simulink model "BESS_test"  (Simulink 8.8)
settings: Solver=ode1  StartTime=0.0  StopTime=15  FixedStep=Ts  MaxStep=1e-3  RelTol=1e-3  EnableMultiTasking=on
model workspace (MAT data in the model file):
  op_snapshot1 : opcond.OperatingPoint (value not decoded)
values from neighbouring files (symbols this model uses):
  dPer = 0.05    [Software_BESS_init.m]
  f = 60    [Software_BESS_init.m]
  filt = firstOrderDig(50e-3, Tc, 'low')    [Software_BESS_init.m]    (also in firstOrderDig.m = (tau*s) / (tau*s + 1))
  H = 2    [Software_BESS_init.m]
  Igrid = Pgrid/Vgrid/3    [Software_BESS_init.m]
  Lgrid = (Zgrid/2)/(2*pi*f)    [Software_BESS_init.m]
  paramDroopFreq2Reac = 0.5*(1/dPer)    (= 10)    [Software_BESS_init.m]
  paramDroopFreq2Real = 0*(1/dPer)    (= 0)    [Software_BESS_init.m]
  paramDroopVolts2Reac = 0*(1/dPer)    (= 0)    [Software_BESS_init.m]
  paramDroopVolts2Real = 0.5*(1/dPer)    (= 10)    [Software_BESS_init.m]
  Pgrid = 3e6    (= 3000000)    [Software_BESS_init.m]
  Rgrid = Zgrid/2    [Software_BESS_init.m]
  sys_mech = ss(1/(tau_mech*s+1))    [Software_BESS_init.m]
  Tc = Ts    (= 0.0001)    [Software_BESS_init.m]
  Ts = 100e-6    (= 0.0001)    [Software_BESS_init.m]
  Vdc_nom = 1000    [Software_BESS_init.m]
  Vgrid = 480/sqrt(3)    [Software_BESS_init.m]
undefined symbols (not defined in the file or in its folder): BESS, BESS_lib, DiscIntNeverNeededParam, RotatingMachine_lib, VSource
undefined symbols (not defined in the file): batt_esr, batt_kWh
libraries: powerlib x29, simulink x7, powerlib_meascontrol x6, transformer_lib x4, breaker_lib x3, Load_lib x3, cables_lib x2, IsourcePower_lib x1
settings Model: ARTEMISmethode_block_infos=$$__separator__$$RS/ARTEMIS Guide$$__separator__$$  Creator=RE25624  LastModifiedBy=ch24070
settings SolverCC: ZeroCrossAlgorithm=Adaptive
settings DataIOCC: ExternalInput=getinputstruct(op_snapshot1)  InitialState=getstatestruct(op_snapshot1)  LimitDataPoints=off  MaxDataPoints=90060  SignalLoggingSaveFormat=Dataset  SaveOutput=off  SignalLogging=off  DSMLogging=off  SaveTime=off  OutputSaveName=result
settings OptimizationCC: BlockReduction=off  OptimizeBlockIOStorage=off  BufferReuse=off  GlobalBufferReuse=off  ExpressionFolding=off  ExpressionDepthLimit=2147483647  LocalBlockOutputs=off  EfficientMapNaN2IntZero=off
settings DebuggingCC: MaxConsecutiveZCsMsg=warning  IgnoredZcDiagnostic=none  MultiTaskRateTransMsg=warning  UnconnectedLineMsg=none  ModelReferenceExtraNoncontSigs=warning
settings HardwareCC: TargetBitPerPointer=64  TargetBitPerSizeT=64  TargetBitPerPtrDiffT=64  TargetLongLongMode=on  TargetIntDivRoundTo=Zero  TargetEndianess=LittleEndian  TargetWordSize=64  TargetHWDeviceType=MATLAB Host  ProdEqTarget=off
settings ModelReferenceCC: UpdateModelReferenceTargets=IfOutOfDate
settings SFSimCC: SFSimEcho=off
settings CodeAppCC: MaxIdLength=128
settings GRTTargetCC: GeneratePreprocessorConditionals=Use local settings

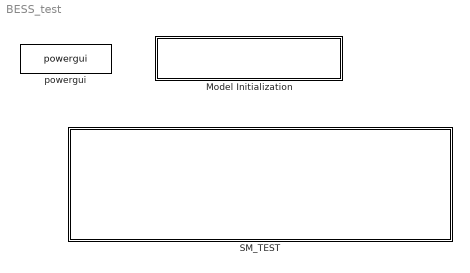
== system BESS_test ==
  Model Initialization : Subsystem  AncestorBlock=artemis/Tools /Misc/Model Initialization  mask(Model Functions){InitFcnX=, prel=off, posl=on, inif=on, strf=off}
      mask prompts: InitFcnX "Initialisation"; prel "Preload Function"; posl "PostLoad Function"; inif "InitFcn"; strf "StartFcn"
      mask init:
      | currentBlock = gcb;
      | root = bdroot(currentBlock);
      | 
      | if ~strcmp(get_param(root,'BlockDiagramType'),'library')
      |     if prel==1
      |         set_param(root, 'PreLoadFcn', InitFcnX);
      |     else
      |         set_param(root, 'PreLoadFcn', '');
      |     end
      |     if inif==1
      |         set_param(root, 'InitFcn', InitFcnX);
      |     else
      |         set_param(root, 'InitFcn', '');
      |     end
      |     if strf==1
      |         set_param(root, 'StartFcn', InitFcnX);
      |     else
      |         set_param(root, 'StartFcn', '');
      |     end
      |     if posl==1
      |         set_param(root, 'PostLoadFcn', InitFcnX);
      |     else
      |         set_param(root, 'PostLoadFcn', '');
      |     end
      | end
      | 
      | pos = get_param(currentBlock, 'Position');
      | width = pos(3) - pos(1); height = pos(4) - pos(2);
      | txt = [ upper(root) '\n' '- InitFcn. . . . . '  get_param(root, 'InitFcn') ];
      settings: CopyFcn=set_param(gcb,'LinkStatus','inactive')
      mask Display: text(5, height*0.5, txt, 'horizontalAlignment', 'left', 'verticalAlignment', 'middle') ;
  SM_TEST : Subsystem
  powergui : powerlib/powergui  Priority=2  SimulationMode=Discrete  SolverType=Tustin  SampleTime=Ts  frequency=60  SPID=off  DisableSnubberDevices=off  DisableRonSwitches=off  DisableVfSwitches=off  SwTol=0  DisplayEquations=off  Interpol=off  ExternalGateDelay=off  methode=off  Ts=0  FunctionMessages=off  echomessages=off  HookPort=off  EnableUseOfTLC=off  x0status=blocks  frequencyindice=0  Pbase=100e6  ErrMax=1e-4  Iterations=50  UnitsV=kV  UnitsW=MW  buscounter=0  RestoreLinks=warning  ResistiveCurrentMeasurement=off  Frange=logspace(-2,3,50)  Ylog=on  Xlog=on  ShowGrid=off  save=off  variable=ZData  structure=0  ZoomFFT=on  StartTime=0.0  cycles=2  DisplayStyle=off  fundamental=60  FreqAxis=off  MaxFrequency=1000  frequencyindicesteady=1  RmsSteady=1  display=off

== system BESS_test/Model Initialization ==

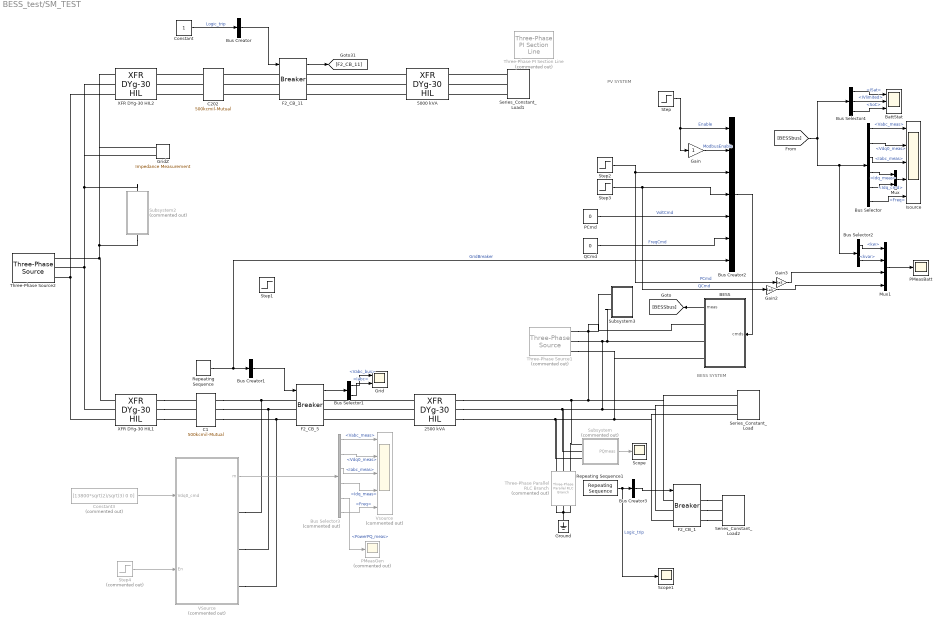
== system BESS_test/SM_TEST ==
  note: PV SYSTEM
  note: BESS SYSTEM
  2500 kVA : transformer_lib/XFR DYg-30 HIL  Rating=2500  Vp=13800  Vs=480  Z=5.56  XR=5.52
  5000 kVA : transformer_lib/XFR DYg-30 HIL  Rating=5000  Vp=13800  Vs=480  Z=5.50  XR=5.44
  BESS : Subsystem  AncestorBlock=BESS_lib/BESS
  BattStat : Scope  NumInputPorts=3
  Bus Creator : BusCreator  Inputs=1
  Bus Creator1 : BusCreator  Inputs=1
  Bus Creator2 : BusCreator  Inputs=7
  Bus Creator3 : BusCreator  Inputs=1
  Bus Selector : BusSelector  OutputSignals=Inverter.Vabc_meas,Inverter.Vdq0_meas,Inverter.Iabc_meas,Inverter.Idq_meas,Inverter.Idq_cmd,Inverter.Freq
  Bus Selector1 : BusSelector  OutputSignals=Vabc_bus,Iabc
  Bus Selector2 : BusSelector  OutputSignals=Inverter.kw,Inverter.kvar
  Bus Selector3 : BusSelector  Commented=on  OutputSignals=Vabc_meas,Vdq0_meas,Iabc_meas,Idq_meas,PowerPQ_meas,Freq
  Bus Selector4 : BusSelector  OutputSignals=Inverter.faults.ISat,Inverter.faults.IVlimited,Battery.SoC
  C1 : cables_lib/500kcmil-Mutual  length=2000  par_sets=1  ratio=3
  C202 : cables_lib/500kcmil-Mutual  length=2000  par_sets=1  ratio=3
  Constant : Constant
  Constant3 : Constant  Commented=on  Value=[13800*sqrt(2)/sqrt(3) 0 0]
  F2_CB_1 : breaker_lib/Breaker  Ts=Ts  mech_delay=3/60
  F2_CB_11 : breaker_lib/Breaker  Ts=Ts  mech_delay=3/60
  F2_CB_5 : breaker_lib/Breaker  Ts=Ts  mech_delay=3/60
  Gain : Gain
  Gain2 : Gain  Gain=1e3
  Gain3 : Gain  Gain=1e3
  Grid : Scope  NumInputPorts=2
  GridZ : powerlib/Measurements/Impedance Measurement  LConnTagsString=+|-  Factor=1
  Ground : powerlib/Elements/Ground  LConnTagsString=a
  Isource : Scope  NumInputPorts=5
  Mux : Mux  Inputs=2
  Mux1 : Mux
  PCmd : Constant  Value=0
  PMeasBatt : Scope
  PMeasGen : Scope  Commented=on
  QCmd : Constant  Value=0
  Repeating Sequence : simulink/Sources/Repeating Sequence  rep_seq_t=[0 2 2+Ts 6 6+Ts 100]  rep_seq_y=[1 1 0 0 1 1]
  Repeating Sequence1 : simulink/Sources/Repeating Sequence  rep_seq_t=[0, 4, 4+Ts, 5, 5+Ts, 8, 8+Ts 20]  rep_seq_y=[0 0 1 1 0 0 1 1]
  Scope : Scope
  Scope1 : Scope
  Series_Constant_Load : Load_lib/Series_Constant_Load  v=460  kVA=400  pf=0.90
  Series_Constant_Load1 : Load_lib/Series_Constant_Load  v=460  kVA=100  pf=0.90
  Series_Constant_Load2 : Load_lib/Series_Constant_Load  v=460  kVA=300  pf=0.90
  Step : Step  Time=0.2  SampleTime=0
  Step1 : Step  Time=0.5  Before=1  After=0  SampleTime=0
  Step2 : Step  Time=9  After=-500  SampleTime=0
  Step3 : Step  Time=13  After=-500  SampleTime=0
  Step4 : Step  Commented=on  Time=0  SampleTime=0
  Subsystem : Subsystem  Commented=on  mask{V=480, P=1e3, PF=0.9}
      mask prompts: V "Nominal voltage LL"; P "P (kVA)"
      mask init:
      | Rpar = V^2/(P*1e3*PF)
      | Lpar = (V^2/((P*1e3*sqrt(1-PF^2))/3))/377
      | if Lpar == Inf
      |     Lser=0
      |     Rser=Rpar
      | else
      |     Lser = 1e-3
      |     Rser = (-Lpar^2)/(Rpar+Lpar)+Lpar-Lser
      | end
  Subsystem2 : Subsystem  Commented=on
  Subsystem3 : Subsystem
  Three-Phase PI Section Line : powerlib/Elements/Three-Phase PI Section Line  Commented=on  LConnTagsString=a|b|c  RConnTagsString=A|B|C  Frequency=60  Resistances=[ 0.01273 0.3864]  Inductances="[ 0.9337e-3  4.1264e-3]"  Capacitances=[12.74e-9 7.751e-9]  Length=100
  Three-Phase Parallel RLC Branch : powerlib/Elements/Three-Phase Parallel RLC Branch  Commented=on  LConnTagsString=A|B|C  RConnTagsString=A|B|C  BranchType=R  Resistance=Vgrid^2/(200*1e3/3);  Inductance=(Vgrid^2/((1000e3*sqrt(1-0.9^2))/3))/377  Capacitance=1e-6  Measurements=None
  Three-Phase Source1 : powerlib/Electrical Sources/Three-Phase Source  Commented=on  InternalConnection=Yg  VoltagePhases=off  Voltage=480  PhaseAngle=0  Voltage_phases=[25e3 25e3 25e3]/sqrt(3)  PhaseAngles_phases=[0 -120 +120]  Frequency=60  NonIdealSource=on  SpecifyImpedance=off  Resistance=Lgrid  Inductance=Rgrid  ShortCircuitLevel=2000e6  BaseVoltage=480  XRratio=100  BusType=swing  Pref=0  Qref=0  Prefabc=[10e3, 10e3, 10e3]  Qrefabc=[0, 0, 0]  Qmin=-inf  Qmax=inf
  Three-Phase Source2 : powerlib/Electrical Sources/Three-Phase Source  InternalConnection=Yg  VoltagePhases=off  Voltage=115000  PhaseAngle=0  Voltage_phases=[25e3 25e3 25e3]/sqrt(3)  PhaseAngles_phases=[0 -120 +120]  Frequency=60  NonIdealSource=on  SpecifyImpedance=on  Resistance=0.8929  Inductance=16.58e-3  ShortCircuitLevel=2000e6  BaseVoltage=115000  XRratio=100  BusType=swing  Pref=0  Qref=0  Prefabc=[10e3, 10e3, 10e3]  Qrefabc=[0, 0, 0]  Qmin=-inf  Qmax=inf
  VSource : Subsystem  Commented=on  AncestorBlock=RotatingMachine_lib/VSource
  Vsource : Scope  Commented=on  NumInputPorts=5
  XFR DYg-30 HIL1 : transformer_lib/XFR DYg-30 HIL  Rating=50000  Vp=115000  Vs=13800  Z=6  XR=30
  XFR DYg-30 HIL2 : transformer_lib/XFR DYg-30 HIL  Rating=50000  Vp=115000  Vs=13800  Z=6  XR=30
  wires:
  F2_CB_5/1 -> Bus Selector1/1
  F2_CB_11/1 -> [F2_CB_11]
  Constant/1 -> Bus Creator/1  "Logic_trip"
  Repeating Sequence/1 -> Bus Creator2/7, Bus Creator1/1  "GridBreaker"
  Bus Creator1/1 -> F2_CB_5/1
  Bus Creator/1 -> F2_CB_11/1
  Step/1 -> Bus Creator2/1, Gain/1  "Enable"
  Step2/1 -> Bus Creator2/3, Gain3/1  "PCmd"
  Step3/1 -> Bus Creator2/4, Gain2/1  "QCmd"
  Bus Creator2/1 -> BESS/1(cmds)
  Bus Selector/6 -> Isource/5  "<Freq>"
  Bus Selector/3 -> Isource/3  "<Iabc_meas>"
  Bus Selector/1 -> Isource/1  "<Vabc_meas>"
  Bus Selector/2 -> Isource/2  "<Vdq0_meas>"
  Subsystem/1(PQmeas) -> Scope/1
  Bus Selector1/1 -> Grid/1  "<Vabc_bus>"
  Bus Selector1/2 -> Grid/2  "<Iabc>"
  Mux/1 -> Isource/4
  Bus Selector/4 -> Mux/1  "<Idq_meas>"
  Bus Selector/5 -> Mux/2  "<Idq_cmd>"
  BESS/1(meas) -> [BESSbus]
  [BESSbus] -> Bus Selector/1, Bus Selector2/1, Bus Selector4/1
  Bus Selector2/1 -> Mux1/1  "<kw>"
  Mux1/1 -> PMeasBatt/1
  Repeating Sequence1/1 -> Scope1/1, Bus Creator3/1  "Logic_trip"
  Bus Creator3/1 -> F2_CB_1/1
  Gain2/1 -> Mux1/4
  Gain3/1 -> Mux1/3
  Constant3/1 -> VSource/1(Vdq0_cmd)
  Step4/1 -> VSource/2(En)
  Bus Selector3/3 -> Vsource/3  "<Iabc_meas>"
  Bus Selector3/1 -> Vsource/1  "<Vabc_meas>"
  Bus Selector3/2 -> Vsource/2  "<Vdq0_meas>"
  Bus Selector3/4 -> Vsource/4  "<Idq_meas>"
  VSource/1(m) -> Bus Selector3/1
  Bus Selector3/6 -> Vsource/5  "<Freq>"
  Bus Selector3/5 -> PMeasGen/1  "<PowerPQ_meas>"
  Gain/1 -> Bus Creator2/2  "ModbusEnable"
  Bus Selector2/2 -> Mux1/2  "<kvar>"
  Bus Selector4/2 -> BattStat/2  "<IVlimited>"
  Bus Selector4/1 -> BattStat/1  "<ISat>"
  Bus Selector4/3 -> BattStat/3  "<SoC>"
  PCmd/1 -> Bus Creator2/5  "VoltCmd"
  QCmd/1 -> Bus Creator2/6  "FreqCmd"
  connections:
  5000 kVA/LConn2 -- F2_CB_11/RConn2
  2500 kVA/LConn1 -- F2_CB_5/RConn1
  2500 kVA/LConn3 -- F2_CB_5/RConn3
  2500 kVA/LConn2 -- F2_CB_5/RConn2
  5000 kVA/LConn1 -- F2_CB_11/RConn1
  5000 kVA/LConn3 -- F2_CB_11/RConn3
  2500 kVA/RConn1 -- BESS/RConn1 -- Subsystem3/LConn1 -- Three-Phase Source1/RConn1 -- F2_CB_1/LConn1 -- Series_Constant_Load/LConn1 -- Three-Phase Parallel RLC Branch/LConn3 -- Subsystem/LConn1
  2500 kVA/RConn3 -- BESS/RConn3 -- Three-Phase Source1/RConn3 -- F2_CB_1/LConn3 -- Series_Constant_Load/LConn3 -- Three-Phase Parallel RLC Branch/LConn1 -- Subsystem/LConn3
  XFR DYg-30 HIL1/LConn1 -- GridZ/LConn1 -- XFR DYg-30 HIL2/LConn1 -- Subsystem2/LConn1 -- Three-Phase Source2/RConn1
  XFR DYg-30 HIL1/LConn2 -- GridZ/LConn2 -- XFR DYg-30 HIL2/LConn2 -- Subsystem2/RConn1 -- Three-Phase Source2/RConn2
  XFR DYg-30 HIL1/LConn3 -- XFR DYg-30 HIL2/LConn3 -- Three-Phase Source2/RConn3
  Series_Constant_Load1/LConn3 -- 5000 kVA/RConn3
  Series_Constant_Load1/LConn2 -- 5000 kVA/RConn2
  Series_Constant_Load1/LConn1 -- 5000 kVA/RConn1
  C202/LConn1 -- XFR DYg-30 HIL2/RConn1
  C202/LConn2 -- XFR DYg-30 HIL2/RConn2
  C202/LConn3 -- XFR DYg-30 HIL2/RConn3
  XFR DYg-30 HIL1/RConn1 -- C1/LConn1
  XFR DYg-30 HIL1/RConn2 -- C1/LConn2
  XFR DYg-30 HIL1/RConn3 -- C1/LConn3
  C1/RConn2 -- VSource/RConn2 -- F2_CB_5/LConn2
  C1/RConn1 -- VSource/RConn1 -- F2_CB_5/LConn1
  C1/RConn3 -- VSource/RConn3 -- F2_CB_5/LConn3
  F2_CB_11/LConn1 -- C202/RConn1
  F2_CB_11/LConn2 -- C202/RConn2
  F2_CB_11/LConn3 -- C202/RConn3
  Ground/LConn1 -- Three-Phase Parallel RLC Branch/RConn3 -- Three-Phase Parallel RLC Branch/RConn1 -- Three-Phase Parallel RLC Branch/RConn2
  F2_CB_1/RConn1 -- Series_Constant_Load2/LConn1
  F2_CB_1/RConn2 -- Series_Constant_Load2/LConn2
  F2_CB_1/RConn3 -- Series_Constant_Load2/LConn3
  Subsystem3/LConn2 -- BESS/RConn2 -- 2500 kVA/RConn2 -- Three-Phase Parallel RLC Branch/LConn2 -- Subsystem/LConn2 -- F2_CB_1/LConn2 -- Series_Constant_Load/LConn2 -- Three-Phase Source1/RConn2

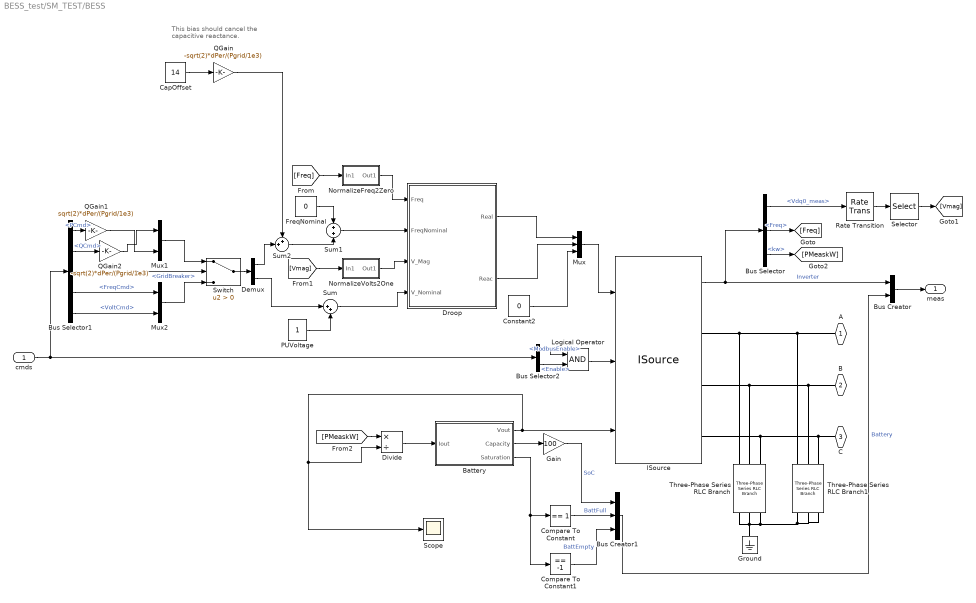
== system BESS_test/SM_TEST/BESS ==
  note: This bias should cancel
      | the capacitive reactance.
  cmds : Inport
  Battery : Subsystem  mask(Very simple battery model.){kWh=batt_kWh, esr=batt_esr, Vdc_nom=Vdc_nom}
      mask prompts: kWh "Capacity  (kWh)"; esr "Output Resistance (Ohms)"; Vdc_nom "Open Circuit Voltage"
      mask help: Model integrates charge and stops at the rated capacity. When charge is all removed the current drops to zero.
      mask Help: This model views the battery as a voltage source with a fixed equivalent series resistance and a perfect integrator for capacity.
  Bus Creator : BusCreator  Inputs=2
  Bus Creator1 : BusCreator  Inputs=3
  Bus Selector : BusSelector  OutputSignals=Vdq0_meas,Freq,kw
  Bus Selector1 : BusSelector  OutputSignals=PCmd,QCmd,GridBreaker,FreqCmd,VoltCmd
  Bus Selector2 : BusSelector  OutputSignals=ModbusEnable,Enable
  CapOffset : Constant  Value=14
  Compare To Constant : simulink/Logic and Bit Operations/Compare To Constant  relop===  const=1  OutDataTypeStr=boolean
  Compare To Constant1 : simulink/Logic and Bit Operations/Compare To Constant  relop===  const=-1  OutDataTypeStr=boolean
  Constant2 : Constant  Value=0
  Demux : Demux  Outputs=2
  Divide : Product  Inputs=*/
  Droop : Subsystem
  FreqNominal : Constant  Value=0
  Gain : Gain  Gain=100
  Ground : powerlib/Elements/Ground  LConnTagsString=a
  ISource : IsourcePower_lib/ISource
  Logical Operator : Logic  AllPortsSameDT=off  OutDataTypeStr=boolean
  Mux : Mux  Inputs=3
  Mux1 : Mux  Inputs=2
  Mux2 : Mux  Inputs=2
  NormalizeFreq2Zero : Subsystem
  NormalizeVolts2One : Subsystem
  PUVoltage : Constant
  QGain : Gain  Gain=-sqrt(2)*dPer/(Pgrid/1e3)
  QGain1 : Gain  Gain=sqrt(2)*dPer/(Pgrid/1e3)
  QGain2 : Gain  Gain=-sqrt(2)*dPer/(Pgrid/1e3)
  Rate Transition : RateTransition  OutPortSampleTime=Tc
  Scope : Scope
  Selector : Selector  InputPortWidth=3  IndexOptions=Index vector (dialog)  Indices=[1]  OutputSizes=1
  Sum : Sum  Inputs=|++
  Sum1 : Sum
  Sum2 : Sum  Inputs=++|
  Switch : Switch  Criteria=u2 > Threshold
  Three-Phase Series RLC Branch : powerlib/Elements/Three-Phase Series RLC Branch  LConnTagsString=A|B|C  RConnTagsString=A|B|C  BranchType=RC  Resistance=10e-3  Inductance=1e-3  Capacitance=1e-3  Measurements=None
  Three-Phase Series RLC Branch1 : powerlib/Elements/Three-Phase Series RLC Branch  LConnTagsString=A|B|C  RConnTagsString=A|B|C  BranchType=R  Resistance=10000  Inductance=1e-3  Capacitance=1000e-9  Measurements=None
  A : PMIOPort  Port=1  Side=Right
  B : PMIOPort  Port=2  Side=Right
  C : PMIOPort  Port=3  Side=Right
  meas : Outport
  wires:
  ISource/1 -> Bus Creator/1, Bus Selector/1  "Inverter"
  cmds/1 -> Bus Selector2/1, Bus Selector1/1
  FreqNominal/1 -> Sum1/1
  Sum/1 -> Droop/4(V_Nominal)
  PUVoltage/1 -> Sum/2
  Sum1/1 -> Droop/2(FreqNominal)
  Constant2/1 -> Mux/3
  [Freq] -> NormalizeFreq2Zero/1(In1)
  Mux/1 -> ISource/1
  Selector/1 -> [Vmag]
  Bus Selector/1 -> Rate Transition/1  "<Vdq0_meas>"
  Bus Selector/2 -> [Freq]  "<Freq>"
  Rate Transition/1 -> Selector/1
  Droop/1(Real) -> Mux/1
  Droop/2(Reac) -> Mux/2
  NormalizeFreq2Zero/1(Out1) -> Droop/1(Freq)
  NormalizeVolts2One/1(Out1) -> Droop/3(V_Mag)
  [Vmag] -> NormalizeVolts2One/1(In1)
  Sum2/1 -> Sum1/2
  QGain/1 -> Sum2/1
  CapOffset/1 -> QGain/1
  Bus Selector2/2 -> Logical Operator/2  "<Enable>"
  Bus Selector2/1 -> Logical Operator/1  "<ModbusEnable>"
  Logical Operator/1 -> ISource/2
  Bus Selector/3 -> [PMeaskW]  "<kw>"
  [PMeaskW] -> Divide/1
  Divide/1 -> Battery/1(Iout)
  Battery/1(Vout) -> ISource/3, Scope/1, Divide/2
  Bus Creator/1 -> meas/1
  Gain/1 -> Bus Creator1/1  "SoC"
  Battery/2(Capacity) -> Gain/1
  Compare To Constant/1 -> Bus Creator1/2  "BattFull"
  Battery/3(Saturation) -> Compare To Constant1/1, Compare To Constant/1
  Compare To Constant1/1 -> Bus Creator1/3  "BattEmpty"
  Bus Creator1/1 -> Bus Creator/2  "Battery"
  Bus Selector1/3 -> Switch/2  "<GridBreaker>"
  Switch/1 -> Demux/1
  Demux/1 -> Sum2/2
  Demux/2 -> Sum/1
  Mux2/1 -> Switch/3
  Bus Selector1/1 -> QGain1/1  "<PCmd>"
  Bus Selector1/2 -> QGain2/1  "<QCmd>"
  Bus Selector1/4 -> Mux2/1  "<FreqCmd>"
  Bus Selector1/5 -> Mux2/2  "<VoltCmd>"
  Mux1/1 -> Switch/1
  QGain1/1 -> Mux1/2
  QGain2/1 -> Mux1/1
  connections:
  Three-Phase Series RLC Branch/LConn1 -- Three-Phase Series RLC Branch1/LConn1 -- A/RConn1 -- ISource/RConn1
  Three-Phase Series RLC Branch/LConn3 -- Three-Phase Series RLC Branch1/LConn3 -- C/RConn1 -- ISource/RConn3
  Three-Phase Series RLC Branch/LConn2 -- Three-Phase Series RLC Branch1/LConn2 -- B/RConn1 -- ISource/RConn2
  Ground/LConn1 -- Three-Phase Series RLC Branch1/RConn3 -- Three-Phase Series RLC Branch1/RConn2 -- Three-Phase Series RLC Branch1/RConn1 -- Three-Phase Series RLC Branch/RConn3 -- Three-Phase Series RLC Branch/RConn1 -- Three-Phase Series RLC Branch/RConn2

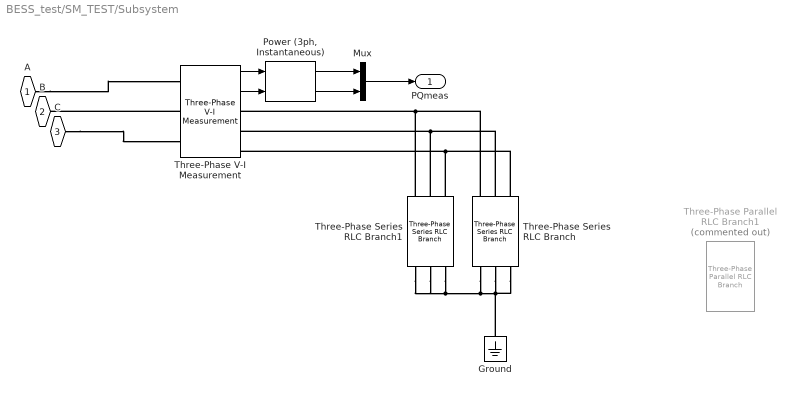
== system BESS_test/SM_TEST/Subsystem ==
  Ground : powerlib/Elements/Ground  LConnTagsString=a
  Mux : Mux  Inputs=2
  "Power (3ph, Instantaneous)" : powerlib_meascontrol/Measurements/Power (3ph, Instantaneous)
  Three-Phase Parallel RLC Branch1 : powerlib/Elements/Three-Phase Parallel RLC Branch  Commented=on  LConnTagsString=A|B|C  RConnTagsString=A|B|C  BranchType=RL  Resistance=Vgrid^2/(1000e3*0.9/3)  Inductance=(Vgrid^2/((1000e3*sqrt(1-0.9^2))/3))/377  Capacitance=1e-6  Measurements=None
  Three-Phase Series RLC Branch : powerlib/Elements/Three-Phase Series RLC Branch  LConnTagsString=A|B|C  RConnTagsString=A|B|C  BranchType=L  Resistance=Rser  Inductance=Lpar  Capacitance=1e-6  Measurements=None
  Three-Phase Series RLC Branch1 : powerlib/Elements/Three-Phase Series RLC Branch  LConnTagsString=A|B|C  RConnTagsString=A|B|C  BranchType=R  Resistance=Rpar  Inductance=Lser  Capacitance=1e-6  Measurements=None
  Three-Phase V-I Measurement : powerlib/Measurements/Three-Phase V-I Measurement  VoltageMeasurement=phase-to-ground  SetLabelV=off  LabelV=Vabc  Vpu=off  VpuLL=off  CurrentMeasurement=yes  SetLabelI=off  LabelI=Iabc  Ipu=off  Pbase=100e6  Vbase=500e3  OutputType=Complex  PhasorSimulation=off  PSBequivalent=0
  A : PMIOPort  Port=1  Side=Left
  B : PMIOPort  Port=2  Side=Left
  C : PMIOPort  Port=3  Side=Left
  PQmeas : Outport
  wires:
  Three-Phase V-I Measurement/1 -> "Power (3ph, Instantaneous)"/1
  Three-Phase V-I Measurement/2 -> "Power (3ph, Instantaneous)"/2
  "Power (3ph, Instantaneous)"/1 -> Mux/1
  "Power (3ph, Instantaneous)"/2 -> Mux/2
  Mux/1 -> PQmeas/1
  connections:
  Three-Phase V-I Measurement/LConn2 -- B/RConn1
  C/RConn1 -- Three-Phase V-I Measurement/LConn3
  A/RConn1 -- Three-Phase V-I Measurement/LConn1
  Three-Phase Series RLC Branch/LConn1 -- Three-Phase Series RLC Branch1/LConn1 -- Three-Phase V-I Measurement/RConn1
  Three-Phase Series RLC Branch/LConn2 -- Three-Phase Series RLC Branch1/LConn2 -- Three-Phase V-I Measurement/RConn2
  Three-Phase Series RLC Branch/LConn3 -- Three-Phase Series RLC Branch1/LConn3 -- Three-Phase V-I Measurement/RConn3
  Ground/LConn1 -- Three-Phase Series RLC Branch1/RConn3 -- Three-Phase Series RLC Branch1/RConn2 -- Three-Phase Series RLC Branch1/RConn1 -- Three-Phase Series RLC Branch/RConn1 -- Three-Phase Series RLC Branch/RConn2 -- Three-Phase Series RLC Branch/RConn3

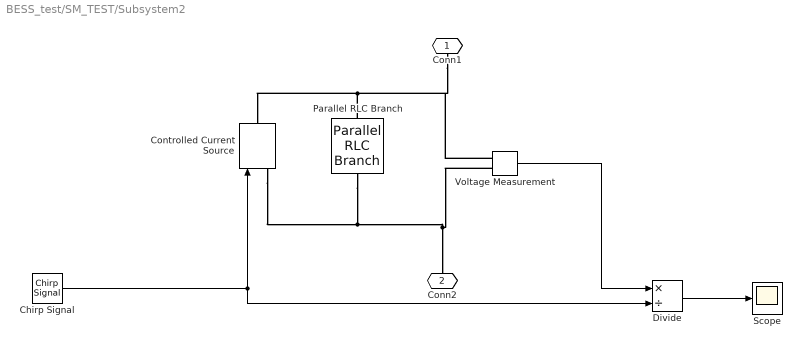
== system BESS_test/SM_TEST/Subsystem2 ==
  Chirp Signal : simulink/Sources/Chirp Signal  f1=0.1  T=1  f2=1000
  Controlled Current Source : powerlib/Electrical Sources/Controlled Current Source  Initialize=on  Source_Type=AC  Amplitude=0  Phase=0  Frequency=0  Measurements=None
  Divide : Product  Inputs=*/
  Parallel RLC Branch : powerlib/Elements/Parallel RLC Branch  LConnTagsString=a  RConnTagsString=__new0  BranchType=R  Resistance=1e6  Inductance=1e-3  SetiL0=off  InitialCurrent=0  Capacitance=1e-6  Setx0=off  InitialVoltage=0  Measurements=None
  Scope : Scope
  Voltage Measurement : powerlib/Measurements/Voltage Measurement  PhasorSimulation=off  OutputType=Complex  PSBequivalent=0
  Conn1 : PMIOPort  Port=1  Side=Right
  Conn2 : PMIOPort  Port=2  Side=Left
  wires:
  Chirp Signal/1 -> Divide/2, Controlled Current Source/1
  Voltage Measurement/1 -> Divide/1
  Divide/1 -> Scope/1
  connections:
  Controlled Current Source/LConn1 -- Parallel RLC Branch/RConn1 -- Voltage Measurement/LConn2 -- Conn2/RConn1
  Parallel RLC Branch/LConn1 -- Conn1/RConn1 -- Voltage Measurement/LConn1 -- Controlled Current Source/RConn1

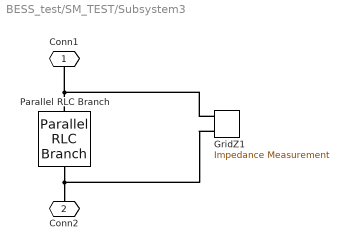
== system BESS_test/SM_TEST/Subsystem3 ==
  GridZ1 : powerlib/Measurements/Impedance Measurement  LConnTagsString=+|-  Factor=1
  Parallel RLC Branch : powerlib/Elements/Parallel RLC Branch  LConnTagsString=a  RConnTagsString=__new0  BranchType=R  Resistance=1e6  Inductance=1e-3  SetiL0=off  InitialCurrent=0  Capacitance=1e-6  Setx0=off  InitialVoltage=0  Measurements=None
  Conn1 : PMIOPort  Port=1  Side=Left
  Conn2 : PMIOPort  Port=2  Side=Left
  connections:
  GridZ1/LConn1 -- Parallel RLC Branch/LConn1 -- Conn1/RConn1
  GridZ1/LConn2 -- Parallel RLC Branch/RConn1 -- Conn2/RConn1

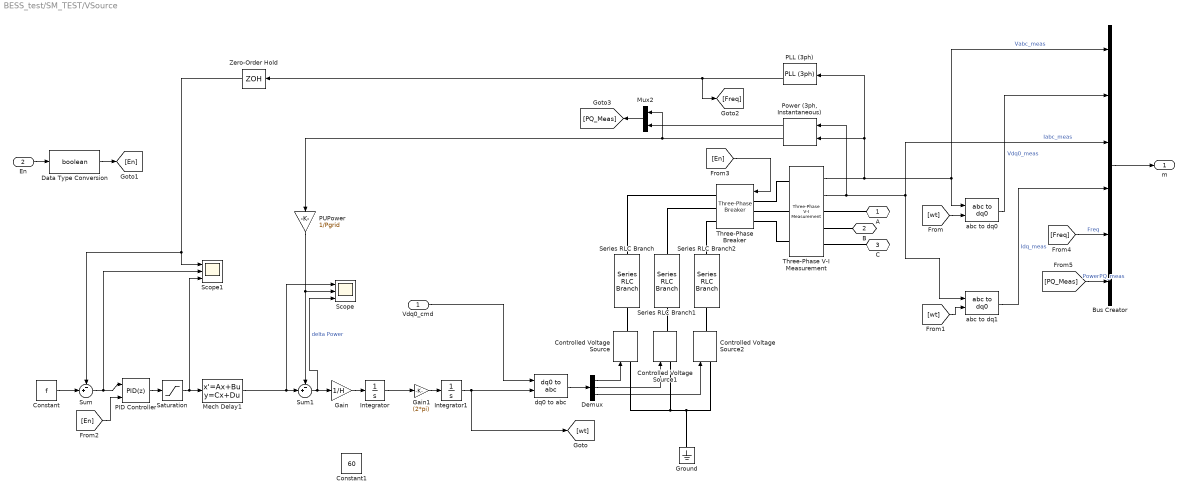
== system BESS_test/SM_TEST/VSource ==
  Vdq0_cmd : Inport
  En : Inport  Port=2
  Bus Creator : BusCreator  Inputs=6
  Constant : Constant  Value=f
  Constant1 : Constant  Value=60
  Controlled Voltage Source : powerlib/Electrical Sources/Controlled Voltage Source  Initialize=on  Source_Type=AC  Amplitude=0  Phase=0  Frequency=0  Measurements=None
  Controlled Voltage Source1 : powerlib/Electrical Sources/Controlled Voltage Source  Initialize=on  Source_Type=AC  Amplitude=0  Phase=0  Frequency=0  Measurements=None
  Controlled Voltage Source2 : powerlib/Electrical Sources/Controlled Voltage Source  Initialize=on  Source_Type=AC  Amplitude=0  Phase=0  Frequency=0  Measurements=None
  Data Type Conversion : DataTypeConversion  OutDataTypeStr=boolean
  Demux : Demux  Outputs=3
  Gain : Gain  Gain=1/H
  Gain1 : Gain  Gain=(2*pi)
  Ground : powerlib/Elements/Ground  LConnTagsString=a
  Integrator : Integrator  InitialCondition=f
  Integrator1 : Integrator
  Mech Delay1 : StateSpace  A=sys_mech.A  B=sys_mech.B  C=sys_mech.C  D=sys_mech.D  X0=0.3/sys_mech.C
  Mux2 : Mux  Inputs=2
  PID Controller : simulink/Continuous/PID Controller  Controller=PID  TimeDomain=Discrete-time  SampleTime=Tc  IntegratorMethod=Forward Euler  FilterMethod=Forward Euler  Form=Parallel  UseFilter=on  ControllerParametersSource=internal  P=10.7070638462033  I=6.52954426447568  D=2.34676955636377  N=24.9126202349528  InitialConditionSource=internal  InitialConditionForIntegrator=0.1  InitialConditionForFilter=0  ExternalReset=level  LimitOutput=off  UpperSaturationLimit=inf  LowerSaturationLimit=-inf  LinearizeAsGain=on  AntiWindupMode=none  Kb=1  TrackingMode=off  Kt=1  PParamMin=[]  PParamMax=[]  IParamMin=[]  IParamMax=[]  DParamMin=[]  DParamMax=[]  NParamMin=[]  NParamMax=[]  KbParamMin=[]  KbParamMax=[]  KtParamMin=[]  KtParamMax=[]  POutMin=[]  POutMax=[]  IOutMin=[]  IOutMax=[]  DOutMin=[]  DOutMax=[]  NOutMin=[]  NOutMax=[]  KbOutMin=[]  KbOutMax=[]  KtOutMin=[]  KtOutMax=[]  IntegratorOutMin=[]  IntegratorOutMax=[]  FilterOutMin=[]  FilterOutMax=[]  SumOutMin=[]  SumOutMax=[]  SumI1OutMin=[]  SumI1OutMax=[]  SumI2OutMin=[]  SumI2OutMax=[]  SumI3OutMin=[]  SumI3OutMax=[]  SumDOutMin=[]  SumDOutMax=[]  SaturationOutMin=[]  SaturationOutMax=[]  IntegratorContinuousStateAttributes=''  IntegratorStateMustResolveToSignalObject=off  IntegratorRTWStateStorageClass=Auto  FilterContinuousStateAttributes=''  FilterStateMustResolveToSignalObject=off  FilterRTWStateStorageClass=Auto  DifferentiatorICPrevScaledInput=0  DifferentiatorOutMin=[]  DifferentiatorOutMax=[]
  PLL (3ph) : powerlib_meascontrol/PLL/PLL (3ph)  Fmin=45  Par_Init=[0, 60]  ParK=[180, 3200, 1]  TcD=1e-4  MaxRateChangeFreq=1200  FilterCutOffFreq=25  Ts=0  AGC=on
  PUPower : Gain  Gain=1/Pgrid
  "Power (3ph, Instantaneous)" : powerlib_meascontrol/Measurements/Power (3ph, Instantaneous)
  Saturation : Saturate  UpperLimit=1.2  LowerLimit=0
  Scope : Scope  NumInputPorts=3
  Scope1 : Scope  NumInputPorts=3
  Series RLC Branch : powerlib/Elements/Series RLC Branch  LConnTagsString=__new0  RConnTagsString=__new0  BranchType=RL  Resistance=Rgrid  Inductance=Lgrid  SetiL0=off  InitialCurrent=0  Capacitance=0  Setx0=off  InitialVoltage=0  Measurements=None
  Series RLC Branch1 : powerlib/Elements/Series RLC Branch  LConnTagsString=__new0  RConnTagsString=__new0  BranchType=RL  Resistance=Rgrid  Inductance=Lgrid  SetiL0=off  InitialCurrent=0  Capacitance=0  Setx0=off  InitialVoltage=0  Measurements=None
  Series RLC Branch2 : powerlib/Elements/Series RLC Branch  LConnTagsString=__new0  RConnTagsString=__new0  BranchType=RL  Resistance=Rgrid  Inductance=Lgrid  SetiL0=off  InitialCurrent=0  Capacitance=0  Setx0=off  InitialVoltage=0  Measurements=None
  Sum : Sum  Inputs=-+|
  Sum1 : Sum  Inputs=-+|
  Three-Phase V-I Measurement : powerlib/Measurements/Three-Phase V-I Measurement  VoltageMeasurement=phase-to-ground  SetLabelV=off  LabelV=Vabc  Vpu=off  VpuLL=off  CurrentMeasurement=yes  SetLabelI=off  LabelI=Iabc  Ipu=off  Pbase=100e6  Vbase=500e3  OutputType=Complex  PhasorSimulation=off  PSBequivalent=0
  Three-Phase Breaker : powerlib/Elements/Three-Phase Breaker  InitialState=open  SwitchA=on  SwitchB=on  SwitchC=on  SwitchTimes="[1/60  5/60]"  External=on  BreakerResistance=0.01  SnubberResistance=1e6  SnubberCapacitance=inf  Measurements=None
  Zero-Order Hold : ZeroOrderHold  SampleTime=Tc
  abc to dq0 : powerlib_meascontrol/Transformations/abc to dq0  Alignment=90 degrees behind phase A axis
  abc to dq1 : powerlib_meascontrol/Transformations/abc to dq0  Alignment=90 degrees behind phase A axis
  dq0 to abc : powerlib_meascontrol/Transformations/dq0 to abc  Alignment=90 degrees behind phase A axis
  A : PMIOPort  Port=1  Side=Right
  B : PMIOPort  Port=2  Side=Right
  C : PMIOPort  Port=3  Side=Right
  m : Outport
  wires:
  Mux2/1 -> [PQ_Meas]
  "Power (3ph, Instantaneous)"/2 -> Mux2/2
  Bus Creator/1 -> m/1
  [Freq] -> Bus Creator/5  "Freq"
  abc to dq0/1 -> Bus Creator/2  "Vdq0_meas"
  Three-Phase V-I Measurement/2 -> abc to dq1/1, Bus Creator/3, "Power (3ph, Instantaneous)"/2  "Iabc_meas"
  Three-Phase V-I Measurement/1 -> abc to dq0/1, Bus Creator/1, "Power (3ph, Instantaneous)"/1, PLL (3ph)/1  "Vabc_meas"
  abc to dq1/1 -> Bus Creator/4  "Idq_meas"
  [PQ_Meas] -> Bus Creator/6  "PowerPQ_meas"
  [En] -> Three-Phase Breaker/1
  [En] -> PID Controller/2
  Data Type Conversion/1 -> [En]
  En/1 -> Data Type Conversion/1
  Constant/1 -> Sum/2
  PUPower/1 -> Sum1/1, Scope/2
  Mech Delay1/1 -> Sum1/2, Scope/1
  PID Controller/1 -> Saturation/1
  Saturation/1 -> Mech Delay1/1, Scope1/3
  Zero-Order Hold/1 -> Scope1/1, Sum/1
  PLL (3ph)/1 -> Zero-Order Hold/1, [Freq]
  Gain1/1 -> Integrator1/1
  "Power (3ph, Instantaneous)"/1 -> PUPower/1, Mux2/1
  Gain/1 -> Integrator/1
  Sum1/1 -> Gain/1, Scope/3  "delta Power"
  Sum/1 -> Scope1/2, PID Controller/1
  Demux/3 -> Controlled Voltage Source2/1
  Demux/2 -> Controlled Voltage Source1/1
  dq0 to abc/1 -> Demux/1
  Demux/1 -> Controlled Voltage Source/1
  Vdq0_cmd/1 -> dq0 to abc/1
  Integrator1/1 -> [wt], dq0 to abc/2
  Integrator/1 -> Gain1/1
  [wt] -> abc to dq0/2
  [wt] -> abc to dq1/2
  connections:
  Three-Phase Breaker/RConn3 -- Series RLC Branch2/LConn1
  Three-Phase Breaker/RConn2 -- Series RLC Branch1/LConn1
  Three-Phase Breaker/RConn1 -- Series RLC Branch/LConn1
  Three-Phase Breaker/LConn3 -- Three-Phase V-I Measurement/LConn3
  Three-Phase Breaker/LConn1 -- Three-Phase V-I Measurement/LConn1
  Three-Phase Breaker/LConn2 -- Three-Phase V-I Measurement/LConn2
  Controlled Voltage Source/LConn1 -- Controlled Voltage Source1/LConn1 -- Controlled Voltage Source2/LConn1 -- Ground/LConn1
  Controlled Voltage Source2/RConn1 -- Series RLC Branch2/RConn1
  Controlled Voltage Source1/RConn1 -- Series RLC Branch1/RConn1
  Controlled Voltage Source/RConn1 -- Series RLC Branch/RConn1
  Three-Phase V-I Measurement/RConn2 -- B/RConn1
  Three-Phase V-I Measurement/RConn1 -- A/RConn1
  Three-Phase V-I Measurement/RConn3 -- C/RConn1

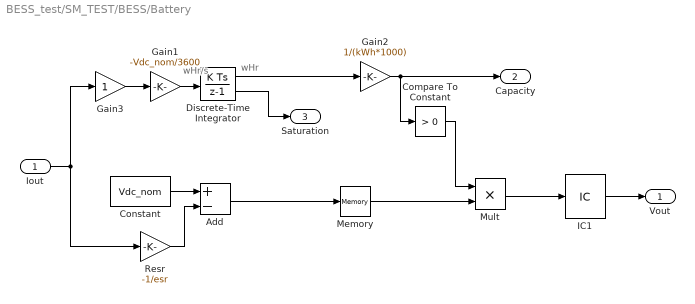
== system BESS_test/SM_TEST/BESS/Battery ==
  note: wHr/s
  note: wHr
  Iout : Inport
  Add : Sum  Inputs=+-
  Compare To Constant : simulink/Logic and Bit Operations/Compare To Constant  relop=>  const=0  OutDataTypeStr=uint8
  Constant : Constant  Value=Vdc_nom  SampleTime=-1
  Discrete-Time Integrator : DiscreteIntegrator  InitialCondition=kWh*0.5*1000  InitialConditionSetting=State (most efficient)  SampleTime=-1  LimitOutput=on  UpperSaturationLimit=kWh*1000  LowerSaturationLimit=0  ShowSaturationPort=on  ICPrevOutput=DiscIntNeverNeededParam  ICPrevScaledInput=DiscIntNeverNeededParam
  Gain1 : Gain  Gain=-Vdc_nom/3600
  Gain2 : Gain  Gain=1/(kWh*1000)
  Gain3 : Gain
  IC1 : InitialCondition  Value=Vdc_nom
  Memory : Memory
  Mult : Product  Inputs=**
  Resr : Gain  Gain=-1/esr
  Vout : Outport
  Capacity : Outport  Port=2
  Saturation : Outport  Port=3
  wires:
  Gain1/1 -> Discrete-Time Integrator/1
  Compare To Constant/1 -> Mult/1
  Mult/1 -> IC1/1
  Iout/1 -> Resr/1, Gain3/1
  Gain2/1 -> Capacity/1, Compare To Constant/1
  Discrete-Time Integrator/1 -> Gain2/1
  IC1/1 -> Vout/1
  Gain3/1 -> Gain1/1
  Discrete-Time Integrator/2 -> Saturation/1
  Constant/1 -> Add/1
  Resr/1 -> Add/2
  Add/1 -> Memory/1
  Memory/1 -> Mult/2

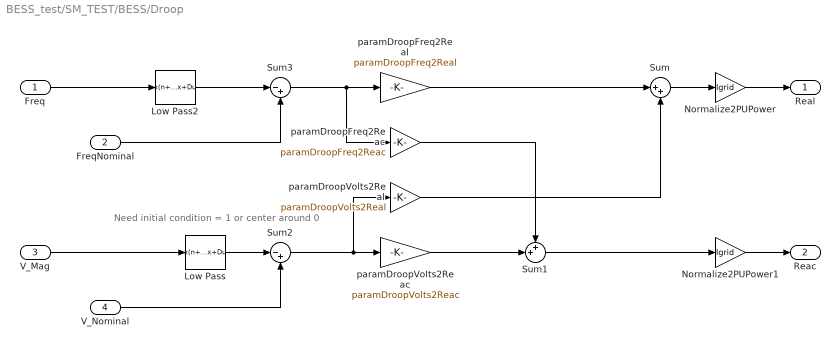
== system BESS_test/SM_TEST/BESS/Droop ==
  note: Need initial condition = 1 or center around 0
  Freq : Inport
  FreqNominal : Inport  Port=2
  V_Mag : Inport  Port=3
  V_Nominal : Inport  Port=4
  Low Pass : DiscreteStateSpace  A=filt.A  B=filt.B  C=filt.C  D=filt.D  X0=1/filt.C  SampleTime=-1
  Low Pass2 : DiscreteStateSpace  A=filt.A  B=filt.B  C=filt.C  D=filt.D  SampleTime=-1
  Normalize2PUPower : Gain  Gain=Igrid
  Normalize2PUPower1 : Gain  Gain=Igrid
  Sum : Sum  Inputs=|++
  Sum1 : Sum  Inputs=++|
  Sum2 : Sum  Inputs=|-+
  Sum3 : Sum  Inputs=|-+
  paramDroopFreq2Reac : Gain  Gain=paramDroopFreq2Reac
  paramDroopFreq2Real : Gain  Gain=paramDroopFreq2Real
  paramDroopVolts2Reac : Gain  Gain=paramDroopVolts2Reac
  paramDroopVolts2Real : Gain  Gain=paramDroopVolts2Real
  Real : Outport
  Reac : Outport  Port=2
  wires:
  V_Mag/1 -> Low Pass/1
  Low Pass2/1 -> Sum3/1
  Sum/1 -> Normalize2PUPower/1
  Sum1/1 -> Normalize2PUPower1/1
  V_Nominal/1 -> Sum2/2
  paramDroopFreq2Real/1 -> Sum/1
  Sum3/1 -> paramDroopFreq2Reac/1, paramDroopFreq2Real/1
  paramDroopVolts2Reac/1 -> Sum1/2
  paramDroopFreq2Reac/1 -> Sum1/1
  Sum2/1 -> paramDroopVolts2Real/1, paramDroopVolts2Reac/1
  paramDroopVolts2Real/1 -> Sum/2
  Low Pass/1 -> Sum2/1
  FreqNominal/1 -> Sum3/2
  Freq/1 -> Low Pass2/1
  Normalize2PUPower/1 -> Real/1
  Normalize2PUPower1/1 -> Reac/1

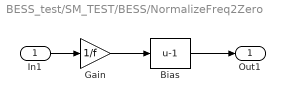
== system BESS_test/SM_TEST/BESS/NormalizeFreq2Zero ==
  In1 : Inport
  Bias : Bias  Bias=-1
  Gain : Gain  Gain=1/f
  Out1 : Outport
  wires:
  Bias/1 -> Out1/1
  In1/1 -> Gain/1
  Gain/1 -> Bias/1

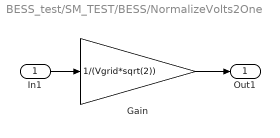
== system BESS_test/SM_TEST/BESS/NormalizeVolts2One ==
  In1 : Inport
  Gain : Gain  Gain=1/(Vgrid*sqrt(2))
  Out1 : Outport
  wires:
  In1/1 -> Gain/1
  Gain/1 -> Out1/1
